simulink model "PACEMAKER_v2"  (R2022b)
settings: Solver=FixedStepAuto  StartTime=0.0  StopTime=10.0  FixedStep=1e-3  RelTol=1e-3  EnableMultiTasking=on
undefined symbols (not defined in the file): D0, D1, D10, D11, D12, D13, D2, D3, D4, D5, D6, D7, D8, D9, PTA0, PTA1, PTA2, PTB23, PTB9, PTC16, PTC17, PTC2, PTC3, PTC4, PTD0, PTD1, PTD2, PTD3
libraries: frdmk64flib x15
settings Model: ExtModeTrigDuration=5  Creator=mutha  LastModifiedBy=jathe
settings SolverCC: AlgebraicLoopSolver=TrustRegion
settings OptimizationCC: EnhancedBackFolding=on  PassReuseOutputArgsAs=Individual arguments  ZeroExternalMemoryAtStartup=off  ZeroInternalMemoryAtStartup=off  MaxStackSize=64  OptimizeBlockOrder=speed  DifferentSizesBufferReuse=on  OptimizationCustomize=off  EfficientTunableParamExpr=on
settings DebuggingCC: ParameterTunabilityLossMsg=error  UnconnectedInputMsg=warning  UnconnectedOutputMsg=warning  UnconnectedLineMsg=warning  SFMachineParentedDataDiag=warning
settings HardwareCC: ProdBitPerPointer=32  ProdBitPerSizeT=32  ProdBitPerPtrDiffT=32  ProdLargestAtomicInteger=Long  ProdLargestAtomicFloat=Double  ProdWordSize=32  ProdHWDeviceType=ARM Compatible->ARM Cortex
settings ModelReferenceCC: EnableRefExpFcnMdlSchedulingChecks=on
settings SFSimCC: MATLABDynamicMemAlloc=off
settings RTWCC: Description=Embedded Coder  SystemTargetFile=ert.tlc  HardwareBoard=NXP FRDM-K64F  TLCOptions="-aInlineSetEventsForThisBaseRateFcn=TLC_FALSE -aSuppressMultiTaskScheduler=TLC_FALSE  -aRateBasedStepFcn=0"  TemplateMakefile=ert_default_tmf  Toolchain=GNU Tools for ARM Embedded Processors  DLArmComputeVersion=19.05
settings CodeAppCC: ForceParamTrailComments=on  IgnoreCustomStorageClasses=off  OperatorAnnotations=on  SimulinkDataObjDesc=on  SFDataObjDesc=on  InsertBlockDesc=on
settings ERTTargetCC: ExtModeTransport=4  ExtModeMexFile=sendToCommService

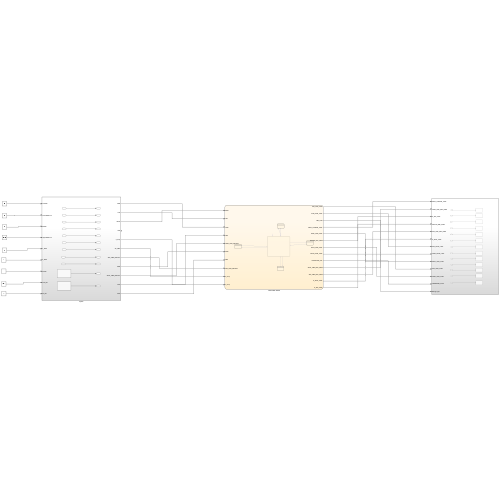
[thumbnail: Simulink's stored preview of the top-level diagram]
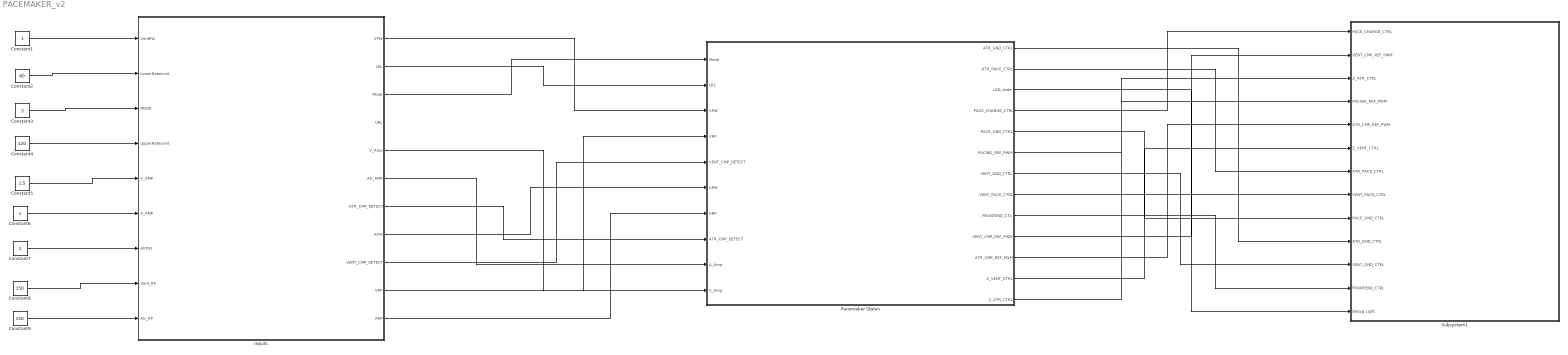
== system PACEMAKER_v2 ==
  Constant1 : Constant  OutDataTypeStr=int16
  Constant2 : Constant  Value=60  OutDataTypeStr=int16
  Constant3 : Constant  Value=3  OutDataTypeStr=int8
  Constant4 : Constant  Value=120  OutDataTypeStr=int16
  Constant5 : Constant  Value=1.5  OutDataTypeStr=double
  Constant6 : Constant  OutDataTypeStr=double
  Constant7 : Constant  OutDataTypeStr=int16
  Constant8 : Constant  Value=150  OutDataTypeStr=int16
  Constant9 : Constant  Value=150  OutDataTypeStr=int16
  Inputs : Subsystem
  Pacemaker States : Stateflow chart  TreatAsAtomicUnit=on
  Subsystem1 : Subsystem
  wires:
  Constant1/1 -> Inputs/1(VentPW)
  Constant2/1 -> Inputs/2(LowerRateLimit)
  Constant3/1 -> Inputs/3(MODE)
  Constant4/1 -> Inputs/4(UpperRateLimit)
  Constant5/1 -> Inputs/5(V_AMP)
  Constant7/1 -> Inputs/7(AtrPW)
  Constant6/1 -> Inputs/6(A_AMP)
  Inputs/3(Mode) -> Pacemaker States/1(Mode)
  Pacemaker States/9(FRONTEND_CTL) -> Subsystem1/12(FRONTEND_CTRL)
  Pacemaker States/1(ATR_GND_CTRL) -> Subsystem1/10(ATR_GND_CTRL)
  Pacemaker States/2(ATR_PACE_CTRL) -> Subsystem1/7(ATR_PACE_CTRL)
  Pacemaker States/3(LED_state) -> Subsystem1/13(Debug Light)
  Pacemaker States/4(PACE_CHARGE_CTRL) -> Subsystem1/1(PACE_CHARGE_CTRL)
  Pacemaker States/5(PACE_GND_CTRL) -> Subsystem1/9(PACE_GND_CTRL)
  Pacemaker States/6(PACING_REF_PWM) -> Subsystem1/4(PACING_REF_PWM)
  Pacemaker States/7(VENT_GND_CTRL) -> Subsystem1/11(VENT_GND_CTRL)
  Pacemaker States/8(VENT_PACE_CTRL) -> Subsystem1/8(VENT_PACE_CTRL)
  Pacemaker States/10(VENT_CMP_REF_PWM) -> Subsystem1/2(VENT_CMP_REF_PWM)
  Pacemaker States/11(ATR_CMP_REF_PWM) -> Subsystem1/5(ATR_CMP_REF_PWM)
  Pacemaker States/12(Z_VENT_CTRL) -> Subsystem1/6(Z_VENT_CTRL)
  Pacemaker States/13(Z_ATR_CTRL) -> Subsystem1/3(Z_ATR_CTRL)
  Inputs/2(LRL) -> Pacemaker States/2(LRL)
  Inputs/7(ATR_CMP_DETECT) -> Pacemaker States/8(ATR_CMP_DETECT)
  Inputs/9(VENT_CMP_DETECT) -> Pacemaker States/5(VENT_CMP_DETECT)
  Inputs/1(VPW) -> Pacemaker States/3(VPW)
  Inputs/8(APW) -> Pacemaker States/6(APW)
  Constant8/1 -> Inputs/8(Vent_RP)
  Constant9/1 -> Inputs/9(Atr_RP)
  Inputs/10(VRP) -> Pacemaker States/4(VRP)
  Inputs/11(ARP) -> Pacemaker States/7(ARP)
  Inputs/5(V_Amp) -> Pacemaker States/10(V_Amp)
  Inputs/6(Atr_AMP) -> Pacemaker States/9(A_Amp)

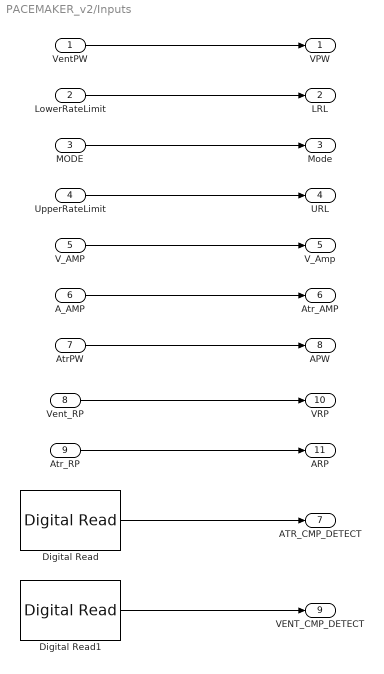
== system PACEMAKER_v2/Inputs ==
  VentPW : Inport  OutDataTypeStr=int16
  LowerRateLimit : Inport  Port=2  OutDataTypeStr=int16
  MODE : Inport  Port=3  OutDataTypeStr=int8
  UpperRateLimit : Inport  Port=4  OutDataTypeStr=int16
  V_AMP : Inport  Port=5  OutDataTypeStr=double
  A_AMP : Inport  Port=6  OutDataTypeStr=double
  AtrPW : Inport  Port=7  OutDataTypeStr=int16
  Vent_RP : Inport  Port=8  OutDataTypeStr=int16
  Atr_RP : Inport  Port=9  OutDataTypeStr=int16
  Digital Read : frdmk64flib/Digital Read  Whichpin=PTC16 (D0)  SampleTime=-1
  Digital Read1 : frdmk64flib/Digital Read  Whichpin=PTC17 (D1)  SampleTime=-1
  VPW : Outport  OutDataTypeStr=int16
  LRL : Outport  Port=2  OutDataTypeStr=int16
  Mode : Outport  Port=3  OutDataTypeStr=int8
  URL : Outport  Port=4  OutDataTypeStr=int16
  V_Amp : Outport  Port=5  OutDataTypeStr=double
  Atr_AMP : Outport  Port=6  OutDataTypeStr=double
  ATR_CMP_DETECT : Outport  Port=7  OutDataTypeStr=boolean
  APW : Outport  Port=8  OutDataTypeStr=int16
  VENT_CMP_DETECT : Outport  Port=9  OutDataTypeStr=boolean
  VRP : Outport  Port=10  OutDataTypeStr=int16
  ARP : Outport  Port=11  OutDataTypeStr=int16
  wires:
  VentPW/1 -> VPW/1
  LowerRateLimit/1 -> LRL/1
  MODE/1 -> Mode/1
  UpperRateLimit/1 -> URL/1
  V_AMP/1 -> V_Amp/1
  A_AMP/1 -> Atr_AMP/1
  AtrPW/1 -> APW/1
  Digital Read/1 -> ATR_CMP_DETECT/1
  Digital Read1/1 -> VENT_CMP_DETECT/1
  Vent_RP/1 -> VRP/1
  Atr_RP/1 -> ARP/1

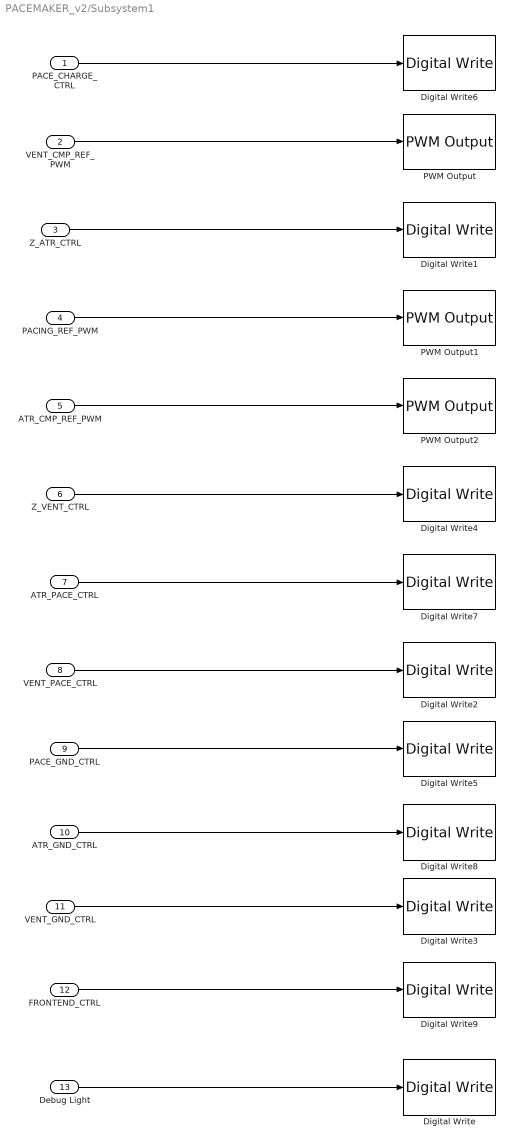
== system PACEMAKER_v2/Subsystem1 ==
  PACE_CHARGE_CTRL : Inport  OutDataTypeStr=boolean
  VENT_CMP_REF_PWM : Inport  Port=2  OutDataTypeStr=double
  Z_ATR_CTRL : Inport  Port=3  OutDataTypeStr=boolean
  PACING_REF_PWM : Inport  Port=4  OutDataTypeStr=double
  ATR_CMP_REF_PWM : Inport  Port=5  OutDataTypeStr=double
  Z_VENT_CTRL : Inport  Port=6  OutDataTypeStr=boolean
  ATR_PACE_CTRL : Inport  Port=7  OutDataTypeStr=boolean
  VENT_PACE_CTRL : Inport  Port=8  OutDataTypeStr=boolean
  PACE_GND_CTRL : Inport  Port=9  OutDataTypeStr=boolean
  ATR_GND_CTRL : Inport  Port=10  OutDataTypeStr=boolean
  VENT_GND_CTRL : Inport  Port=11  OutDataTypeStr=boolean
  FRONTEND_CTRL : Inport  Port=12  OutDataTypeStr=boolean
  Debug Light : Inport  Port=13  OutDataTypeStr=boolean
  Digital Write : frdmk64flib/Digital Write  Whichpin=RED_LED
  Digital Write1 : frdmk64flib/Digital Write  Whichpin=PTB23 (D4)
  Digital Write2 : frdmk64flib/Digital Write  Whichpin=PTC4 (D9)
  Digital Write3 : frdmk64flib/Digital Write  Whichpin=PTD3 (D12)
  Digital Write4 : frdmk64flib/Digital Write  Whichpin=PTC3 (D7)
  Digital Write5 : frdmk64flib/Digital Write  Whichpin=PTD0 (D10)
  Digital Write6 : frdmk64flib/Digital Write  Whichpin=PTB9 (D2)
  Digital Write7 : frdmk64flib/Digital Write  Whichpin=PTA0 (D8)
  Digital Write8 : frdmk64flib/Digital Write  Whichpin=PTD2 (D11)
  Digital Write9 : frdmk64flib/Digital Write  Whichpin=PTD1 (D13)
  PWM Output : frdmk64flib/PWM Output  Whichpin=PTA1 (D3)  InitialFrequency=2000  InitialDutyCycle=0
  PWM Output1 : frdmk64flib/PWM Output  Whichpin=PTA2 (D5)  InitialFrequency=2000  InitialDutyCycle=0
  PWM Output2 : frdmk64flib/PWM Output  Whichpin=PTC2 (D6)  InitialFrequency=2000  InitialDutyCycle=0
  wires:
  VENT_PACE_CTRL/1 -> Digital Write2/1
  VENT_GND_CTRL/1 -> Digital Write3/1
  ATR_GND_CTRL/1 -> Digital Write8/1
  ATR_PACE_CTRL/1 -> Digital Write7/1
  PACE_CHARGE_CTRL/1 -> Digital Write6/1
  PACING_REF_PWM/1 -> PWM Output1/1
  PACE_GND_CTRL/1 -> Digital Write5/1
  Debug Light/1 -> Digital Write/1
  VENT_CMP_REF_PWM/1 -> PWM Output/1
  Z_ATR_CTRL/1 -> Digital Write1/1
  ATR_CMP_REF_PWM/1 -> PWM Output2/1
  Z_VENT_CTRL/1 -> Digital Write4/1
  FRONTEND_CTRL/1 -> Digital Write9/1

== stateflow chart PACEMAKER_v2/Pacemaker States ==
  state AOO1
    state LED_on%State2(AOO)
      %Discharging C22
      PACE_CHARGE_CTRL = false;
      PACE_GND_CTRL = true;
      VENT_PACE_CTRL = false;
      ATR_PACE_CTRL = true;
      VENT_GND_CTRL = true; %not sure
      ATR_GND_CTRL = false;
      %LED STATE
      LED_state = true;
    state LED_off %State 1(AOO)
      %Charging C22
      PACING_REF_PWM = (A_Amp / 5)*100;
      PACE_CHARGE_CTRL = true;
      VENT_PACE_CTRL = false;
      ATR_PACE_CTRL = false;
      %Discharging C21
      PACE_GND_CTRL = true;
      VENT_GND_CTRL = false;
      ATR_GND_CTRL = true;
      %LED STATE
      LED_state = false;
    LED_off %State 1(AOO) -> 77 [order 1] : [Mode~=2]
    (default) -> LED_off %State 1(AOO)
    LED_off %State 1(AOO) -> LED_on%State2(AOO) [order 2] : after ((60000/LRL) - APW, msec)
    LED_on%State2(AOO) -> LED_off %State 1(AOO) : after (APW,msec)
  state Start_State %Default Start State
    entry:
    VENT_PACE_CTRL = false;
    ATR_PACE_CTRL = false;
    VENT_GND_CTRL = false;
    ATR_GND_CTRL = false;
    PACE_GND_CTRL = false;
    PACE_CHARGE_CTRL = false;
    FRONTEND_CTL = false;
    VENT_CMP_REF_PWM = 0;
    PACING_REF_PWM = 0;
    ATR_CMP_REF_PWM = 0;
    Z_ATR_CTRL = false;
    Z_VENT_CTRL = false;
  state VOO1
    state LED_off %State 1(VOO)
      entry:
      %Charging C22
      PACING_REF_PWM = (V_Amp / 5)*100;
      PACE_CHARGE_CTRL = true;
      VENT_PACE_CTRL = false;
      ATR_PACE_CTRL = false;
      %Discharging C21
      PACE_GND_CTRL = true;
      VENT_GND_CTRL = true;
      ATR_GND_CTRL = false;
      %LED STATE
      LED_state = false;
    state LED_on%State2(VOO)
      entry:
      %Discharging C22
      PACE_CHARGE_CTRL = false;
      PACE_GND_CTRL = true;
      VENT_PACE_CTRL = true;
      ATR_PACE_CTRL = false;
      VENT_GND_CTRL = false;
      ATR_GND_CTRL = true; %not sure
      %LED STATE
      LED_state = true;
    LED_off %State 1(VOO) -> 88 [order 1] : [Mode ~= 1]
    (default) -> LED_off %State 1(VOO)
    LED_off %State 1(VOO) -> LED_on%State2(VOO) [order 2] : after ((60000/LRL) - VPW, msec)
    LED_on%State2(VOO) -> LED_off %State 1(VOO) : after (VPW,msec)
  state AAI1
    state SENSE_PULSE %Start sensing after ARP
      entry:
      LED_state = true;
    state SETUP_ATR_SENSE %State 1(VOO)
      entry:
      FRONTEND_CTL = true;
      ATR_CMP_REF_PWM = 52;
      PACING_REF_PWM = (A_Amp / 5)*100;
      PACE_CHARGE_CTRL = true;
      VENT_PACE_CTRL = false;
      ATR_PACE_CTRL = false;
      %Discharging C21
      PACE_GND_CTRL = true;
      VENT_GND_CTRL = false;
      ATR_GND_CTRL = true;
      %LED STATE
      LED_state = false;
    state ATR_PACE_PT2 %Discharging C22
      entry:
      PACE_CHARGE_CTRL = false;
      ATR_PACE_CTRL = true;
      ATR_GND_CTRL = false;
      %LED STATE
      LED_state = true;
    SETUP_ATR_SENSE %State 1(VOO) -> 118 [order 1] : [Mode~=4]
    (default) -> SETUP_ATR_SENSE %State 1(VOO)
    SETUP_ATR_SENSE %State 1(VOO) -> SENSE_PULSE %Start sensing after ARP [order 2] : after(ARP, msec)
    SENSE_PULSE %Start sensing after ARP -> SETUP_ATR_SENSE %State 1(VOO) [order 2] : [ATR_CMP_DETECT==true]
    SENSE_PULSE %Start sensing after ARP -> ATR_PACE_PT2 %Discharging C22 [order 1] : after(60000/LRL - ARP-APW,msec)
    ATR_PACE_PT2 %Discharging C22 -> SETUP_ATR_SENSE %State 1(VOO) : after(APW, msec)
  state VVI1
    state SETUP_VENT_SENSE %State 1(VOO)
      entry:
      FRONTEND_CTL = true;
      VENT_CMP_REF_PWM = 53;
      PACING_REF_PWM = (V_Amp / 5)*100;
      PACE_CHARGE_CTRL = true;
      VENT_PACE_CTRL = false;
      ATR_PACE_CTRL = false;
      %Discharging C21
      PACE_GND_CTRL = true;
      VENT_GND_CTRL = true;
      ATR_GND_CTRL = false;
      %LED STATE
      LED_state = false;
    state SENSE_PULSE %Start sensing after VRP
      entry:
      LED_state=true;
    state VENT_PACE_PT2 %Discharging C22
      entry:
      PACE_CHARGE_CTRL = false;
      PACE_GND_CTRL = true;
      VENT_PACE_CTRL = true;
      ATR_PACE_CTRL = false;
      VENT_GND_CTRL = false; %not sure
      ATR_GND_CTRL = false;
      %LED STATE
      LED_state = true;
    (default) -> SETUP_VENT_SENSE %State 1(VOO)
    SETUP_VENT_SENSE %State 1(VOO) -> 103 [order 1] : [Mode~=3]
    SETUP_VENT_SENSE %State 1(VOO) -> SENSE_PULSE %Start sensing after VRP [order 2] : after(VRP, msec)
    SENSE_PULSE %Start sensing after VRP -> SETUP_VENT_SENSE %State 1(VOO) [order 2] : [VENT_CMP_DETECT==true]
    SENSE_PULSE %Start sensing after VRP -> VENT_PACE_PT2 %Discharging C22 [order 1] : [after(60000/LRL - VRP-VPW, msec)]
    VENT_PACE_PT2 %Discharging C22 -> SETUP_VENT_SENSE %State 1(VOO) : after(VPW,msec)
  Start_State %Default Start State -> AOO1 [order 1] : [Mode==2]
  81 -> Start_State %Default Start State
  (default) -> Start_State %Default Start State
  Start_State %Default Start State -> VOO1 [order 2] : [Mode==1]
  92 -> Start_State %Default Start State
  126 -> Start_State %Default Start State
  Start_State %Default Start State -> AAI1 [order 4] : [Mode==4]
  108 -> Start_State %Default Start State
  Start_State %Default Start State -> VVI1 [order 3] : [Mode==3]
  data: Mode input int8; ATR_GND_CTRL output boolean; ATR_PACE_CTRL output boolean; LED_state output boolean; PACE_CHARGE_CTRL output boolean; PACE_GND_CTRL output boolean; PACING_REF_PWM output double; VENT_GND_CTRL output boolean; VENT_PACE_CTRL output boolean; LRL input int16; FRONTEND_CTL output boolean; VENT_CMP_REF_PWM output double; VPW input int16; VRP input int16; VENT_CMP_DETECT input boolean; ATR_CMP_REF_PWM output double; APW input int16; ARP input int16; ATR_CMP_DETECT input boolean; Z_VENT_CTRL output boolean; Z_ATR_CTRL output boolean; A_Amp input double; V_Amp input double
